simulink model "ref4_rt"  (Simulink 10.0)
settings: Solver=FixedStepDiscrete  StartTime=0.0  StopTime=inf  FixedStep=Ts  RelTol=1e-3  EnableMultiTasking=on
undefined symbols (not defined in the file): Ts
libraries: motion x3, simulink3 x1
settings Model: Creator=bhisma  LastModifiedBy=bhisma
settings DataIOCC: LimitDataPoints=on  MaxDataPoints=10000  SignalLoggingSaveFormat=ModelDataLogs  SaveTime=off
settings OptimizationCC: BlockReduction=off  BooleanDataType=off  LifeSpan=auto
settings DebuggingCC: SaveWithParameterizedLinksMsg=none  SignalResolutionControl=TryResolveAllWithWarning  MultiTaskDSMMsg=warning  MultiTaskCondExecSysMsg=none  SFUnexpectedBacktrackingDiag=error  SFNoUnconditionalDefaultTransitionDiag=error  SFExecutionAtInitializationDiag=warning  ArithmeticOperatorsInVariantConditions=error
settings HardwareCC: ProdBitPerPointer=64  ProdBitPerSizeT=64  ProdBitPerPtrDiffT=64  ProdLargestAtomicFloat=Float  ProdIntDivRoundTo=Zero  ProdEndianess=LittleEndian  ProdWordSize=64  ProdHWDeviceType=Intel->x86-64 (Windows64)  TargetUnknown=on
settings SFSimCC: SimUseLocalCustomCode=on  CustomCodeUndefinedFunction=FilterOut
settings RTWCC: RTWUseLocalCustomCode=on
settings CodeAppCC: StateflowObjectComments=off
settings GRTTargetCC: TargetLangStandard=C99 (ISO)
settings ConfigComp: CovMetricSettings=dwe  CovSaveCumulativeToWorkspaceVar=off  CovSaveSingleToWorkspaceVar=off

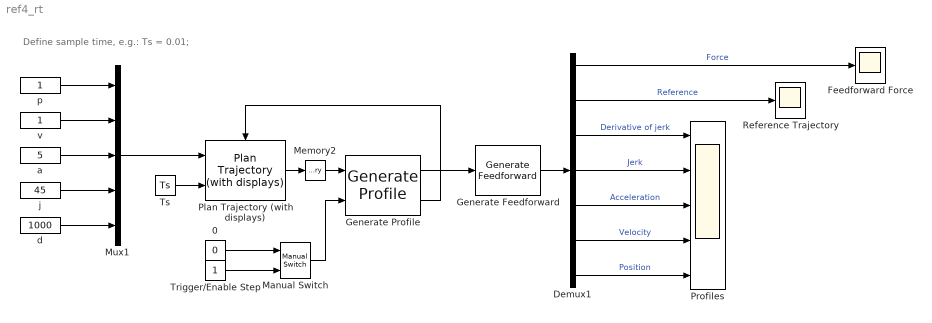
== system ref4_rt ==
  note: Define sample time, e.g.: Ts = 0.01;
  0 : Constant  Value=0
  Demux1 : Demux  Outputs=7
  Feedforward Force : Scope
  Generate Feedforward : motion/Real Time/Generate Feedforward  m1=20  m2=10  k1=10  k2=10  c=6e5  k12=500  Ts=Ts  S1=1  S2=1
  Generate Profile : motion/Real Time/Generate Profile  Ts=Ts  Tset=1
  Manual Switch : simulink3/Nonlinear/Manual Switch  sw=0  action=0
      settings: SourceProductName=Simulink  SourceProductBaseCode=SL
  Memory2 : Memory  InheritSampleTime=on
  Mux1 : Mux  Inputs=5
  Plan Trajectory (with displays) : motion/Real Time/Plan Trajectory (with displays)  TreatAsAtomicUnit=on
      settings: RTWFcnNameOpts=Auto  RTWFileNameOpts=Auto
  Profiles : Scope  NumInputPorts=5
  Reference Trajectory : Scope
  Trigger/Enable Step : Constant
  Ts : Constant  Value=Ts
  a : Constant  Value=5
  d : Constant  Value=1000
  j : Constant  Value=45
  p : Constant
  v : Constant
  wires:
  v/1 -> Mux1/2
  a/1 -> Mux1/3
  j/1 -> Mux1/4
  d/1 -> Mux1/5
  p/1 -> Mux1/1
  Demux1/1 -> Feedforward Force/1  "Force"
  Demux1/2 -> Reference Trajectory/1  "Reference"
  Demux1/3 -> Profiles/1  "Derivative of jerk"
  Demux1/4 -> Profiles/2  "Jerk"
  Demux1/5 -> Profiles/3  "Acceleration"
  Demux1/6 -> Profiles/4  "Velocity"
  Demux1/7 -> Profiles/5  "Position"
  Plan Trajectory (with displays)/1 -> Memory2/1
  Memory2/1 -> Generate Profile/1
  Generate Profile/2 -> Plan Trajectory (with displays)/Trigger
  Generate Profile/1 -> Generate Feedforward/1
  Generate Feedforward/1 -> Demux1/1
  Manual Switch/1 -> Generate Profile/2
  Trigger/Enable Step/1 -> Manual Switch/2
  0/1 -> Manual Switch/1
  Mux1/1 -> Plan Trajectory (with displays)/1
  Ts/1 -> Plan Trajectory (with displays)/2
